simulink model "lab_3"  (Simulink 7.3)
settings: Solver=ode3  StartTime=0  StopTime=100  FixedStep=0.001  RelTol=1e-3
settings Model: Creator=torres.g  LastModifiedBy=torres.g

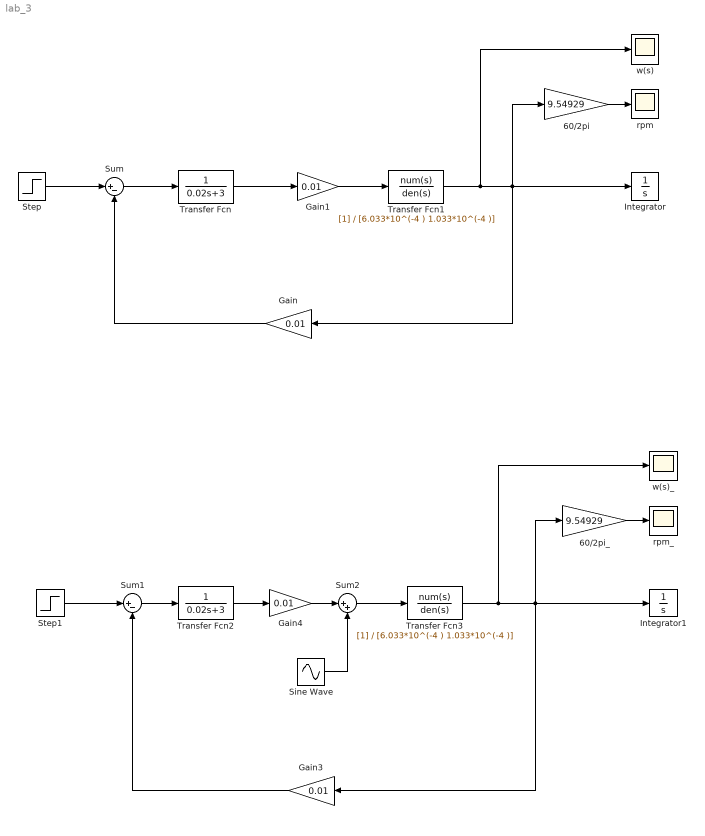
== system lab_3 ==
  60/2pi : Gain  Gain=9.54929  ParameterDataType=fixdt(1, 16)  ParameterScaling=2^0  OutDataType=fixdt(1, 16)  OutScaling=2^0
  60/2pi_ : Gain  Gain=9.54929  ParameterDataType=fixdt(1, 16)  ParameterScaling=2^0  OutDataType=fixdt(1, 16)  OutScaling=2^0
  Gain{,1,3..4} (4 alike) : Gain  Gain=0.01  ParameterDataType=fixdt(1, 16)  ParameterScaling=2^0  OutDataType=fixdt(1, 16)  OutScaling=2^0
  Integrator : Integrator
  Integrator1 : Integrator
  Sine Wave : Sin  Amplitude=0.01  Bias=0  Frequency=1  Phase=0  Samples=10  SampleTime=0  Offset=0
  Step : Step  Time=0  After=12  SampleTime=0
  Step1 : Step  Time=0  After=12  SampleTime=0
  Sum : Sum  Inputs=|+-  OutDataType=fixdt(1, 16)  OutScaling=2^0
  Sum1 : Sum  Inputs=|+-  OutDataType=fixdt(1, 16)  OutScaling=2^0
  Sum2 : Sum  Inputs=|++  OutDataType=fixdt(1, 16)  OutScaling=2^0
  Transfer Fcn : TransferFcn  Denominator=[0.02 3]
  Transfer Fcn1 : TransferFcn  Denominator=[6.033*10^(-4 ) 1.033*10^(-4 )]
  Transfer Fcn2 : TransferFcn  Denominator=[0.02 3]
  Transfer Fcn3 : TransferFcn  Denominator=[6.033*10^(-4 ) 1.033*10^(-4 )]
  rpm : Scope
  rpm_ : Scope
      settings: SaveName=ScopeData2
  w(s) : Scope
  w(s)_ : Scope
      settings: SaveName=ScopeData3
  wires:
  Step/1 -> Sum/1
  Sum/1 -> Transfer Fcn/1
  Transfer Fcn/1 -> Gain1/1
  Gain1/1 -> Transfer Fcn1/1
  Transfer Fcn1/1 -> w(s)/1, Integrator/1, 60/2pi/1, Gain/1
  Gain/1 -> Sum/2
  60/2pi/1 -> rpm/1
  Step1/1 -> Sum1/1
  Sum1/1 -> Transfer Fcn2/1
  Transfer Fcn2/1 -> Gain4/1
  Transfer Fcn3/1 -> w(s)_/1, Integrator1/1, 60/2pi_/1, Gain3/1
  Gain3/1 -> Sum1/2
  60/2pi_/1 -> rpm_/1
  Gain4/1 -> Sum2/1
  Sum2/1 -> Transfer Fcn3/1
  Sine Wave/1 -> Sum2/2
